simulink model "Nordic_2016a"  (R2016a)
settings: Solver=VariableStepAuto  StartTime=0.0  StopTime=600  RelTol=1e-3
values from neighbouring files (symbols this model uses):
  D = 10    [init_nordic.m]    (also in init_shj.m = 50)
  DC = [Y_11-Y_12*X*Y_21 Y_12*X]    [init_nordic.m]
  f0 = 50    [init_nordic.m]    (also in init_shj.m)
  H = [3.592 4.602 3.3 3.558 4.925 3.5 3.494 5.403 3.370 7]    [init_nordic.m]    (also in init_shj.m = 3)
  Kd1 = 0    [init_nordic.m]
  Kp = 2.5    [PID_parameters.m]    (also in init_nordic.m = 2)
  M1 = 5000    [init_nordic.m]    (also in init_shj.m = 300)
  M10 = 7800    [init_nordic.m]
  M2 = 6000    [init_nordic.m]    (also in init_shj.m = 30000)
  M3 = 8000    [init_nordic.m]
  M4 = 4400    [init_nordic.m]
  M5 = 14502    [init_nordic.m]
  M6 = 8000    [init_nordic.m]
  M7 = 2650    [init_nordic.m]
  M8 = 15300    [init_nordic.m]
  M9 = 11000    [init_nordic.m]
  Pl1 = 0    [init_nordic.m]
  Pl10 = 0    [init_nordic.m]
  Pl11 = 0    [init_nordic.m]
  Pl2 = 0    [init_nordic.m]
  Pl3 = 0    [init_nordic.m]
  Pl4 = 0    [init_nordic.m]
  Pl5 = 0    [init_nordic.m]
  Pl6 = 0    [init_nordic.m]
  Pl7 = 0.7    [init_nordic.m]
  Pl8 = 0    [init_nordic.m]
  Pl9 = 0    [init_nordic.m]
  R1 = 0.12    [init_nordic.m]
  R10 = 0.5    [init_nordic.m]
  R2 = R    (= 0.06)    [PID_parameters.m]    (also in init_nordic.m = 0.12)
  R3 = 0.12    [init_nordic.m]
  R4 = 0.12    [init_nordic.m]
  R5 = 0.25    [init_nordic.m]
  R6 = 0.12    [init_nordic.m]
  R7 = 0.12    [init_nordic.m]
  R8 = 0.5    [init_nordic.m]
  R9 = 0.12    [init_nordic.m]
  S_base = 1000    [init_nordic.m]    (also in init_shj.m = 30300)
  Td = 0.6    [PID_parameters.m]    (also in init_nordic.m = 0)
  Tf = 0.2    [PID_parameters.m]    (also in init_nordic.m = 0)
  Ti = 5    [PID_parameters.m]    (also in init_nordic.m)
  Tw = 1.5/2    (= 0.75)    [init_nordic.m]    (also in init_shj.m = 1.2)
  Ty = 0    [init_nordic.m]    (also in init_shj.m = 0.2)
  Ysp = 0    [init_nordic.m]    (also in init_shj.m)
settings Model: Creator=sigurd  LastModifiedBy=sigurdja

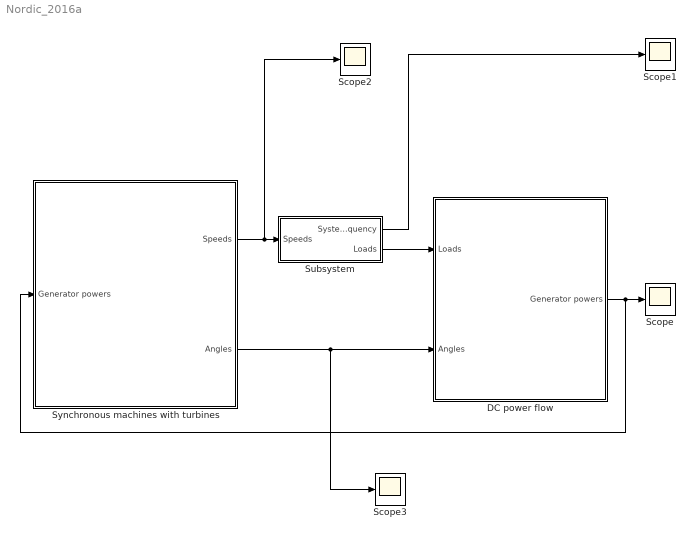
== system Nordic_2016a ==
  DC power flow : Subsystem
  Scope{,1..3} (4 alike) : Scope
  Subsystem : Subsystem
  Synchronous machines with turbines : Subsystem
  wires:
  DC power flow/1(Generator powers) -> Synchronous machines with turbines/1(Generator powers), Scope/1
  Synchronous machines with turbines/1(Speeds) -> Scope2/1, Subsystem/1(Speeds)
  Subsystem/2(Loads) -> DC power flow/1(Loads)
  Synchronous machines with turbines/2(Angles) -> Scope3/1, DC power flow/2(Angles)
  Subsystem/1(System frequency) -> Scope1/1

== system Nordic_2016a/DC power flow ==
  Loads : Inport
  Angles : Inport  Port=2
  Constant : Constant  Value=DC  VectorParams1D=off
  Demux : Demux  Outputs=10
  Demux1 : Demux  Outputs=11
  Gain : Gain  Gain=-1
  Mux : Mux  Inputs=21
  Product : Product  Multiplication=Matrix(*)
  Generator powers : Outport
  wires:
  Product/1 -> Generator powers/1
  Constant/1 -> Product/1
  Angles/1 -> Demux/1
  Loads/1 -> Gain/1
  Demux/1 -> Mux/1
  Demux/2 -> Mux/2
  Demux/3 -> Mux/3
  Demux/4 -> Mux/4
  Demux/5 -> Mux/5
  Demux/6 -> Mux/6
  Demux/7 -> Mux/7
  Demux/8 -> Mux/8
  Demux/9 -> Mux/9
  Demux/10 -> Mux/10
  Demux1/1 -> Mux/11
  Demux1/2 -> Mux/12
  Demux1/3 -> Mux/13
  Demux1/4 -> Mux/14
  Demux1/5 -> Mux/15
  Demux1/6 -> Mux/16
  Demux1/7 -> Mux/17
  Demux1/8 -> Mux/18
  Demux1/9 -> Mux/19
  Demux1/10 -> Mux/20
  Demux1/11 -> Mux/21
  Mux/1 -> Product/2
  Gain/1 -> Demux1/1

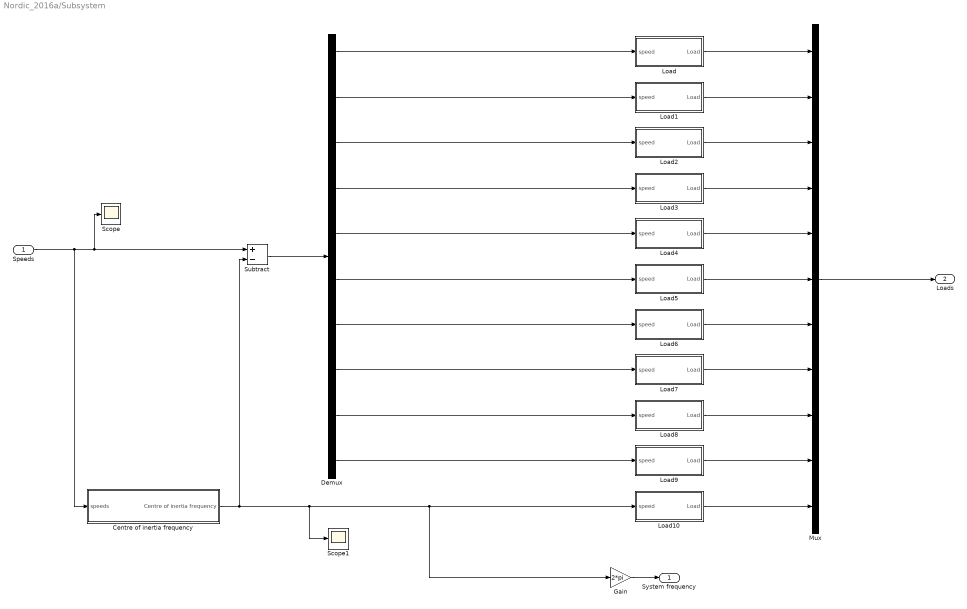
== system Nordic_2016a/Subsystem ==
  Speeds : Inport
  Centre of inertia frequency : Subsystem
  Demux : Demux  Outputs=10
  Gain : Gain  Gain=2*pi
  Load : Subsystem
  Load1 : Subsystem
  Load10 : Subsystem
  Load2 : Subsystem
  Load3 : Subsystem
  Load4 : Subsystem
  Load5 : Subsystem
  Load6 : Subsystem
  Load7 : Subsystem
  Load8 : Subsystem
  Load9 : Subsystem
  Mux : Mux  Inputs=11
  Scope : Scope
  Scope1 : Scope
  Subtract : Sum  Inputs=+-
  System frequency : Outport
  Loads : Outport  Port=2
  wires:
  Speeds/1 -> Centre of inertia frequency/1(speeds), Scope/1, Subtract/1
  Load/1(Load) -> Mux/1
  Load1/1(Load) -> Mux/2
  Load2/1(Load) -> Mux/3
  Load3/1(Load) -> Mux/4
  Load4/1(Load) -> Mux/5
  Load6/1(Load) -> Mux/7
  Load5/1(Load) -> Mux/6
  Load7/1(Load) -> Mux/8
  Load8/1(Load) -> Mux/9
  Mux/1 -> Loads/1
  Load9/1(Load) -> Mux/10
  Load10/1(Load) -> Mux/11
  Gain/1 -> System frequency/1
  Centre of inertia frequency/1(Centre of inertia frequency) -> Subtract/2, Scope1/1, Load10/1(speed), Gain/1
  Subtract/1 -> Demux/1
  Demux/1 -> Load/1(speed)
  Demux/2 -> Load1/1(speed)
  Demux/3 -> Load2/1(speed)
  Demux/4 -> Load3/1(speed)
  Demux/5 -> Load4/1(speed)
  Demux/6 -> Load5/1(speed)
  Demux/7 -> Load6/1(speed)
  Demux/8 -> Load7/1(speed)
  Demux/9 -> Load8/1(speed)
  Demux/10 -> Load9/1(speed)

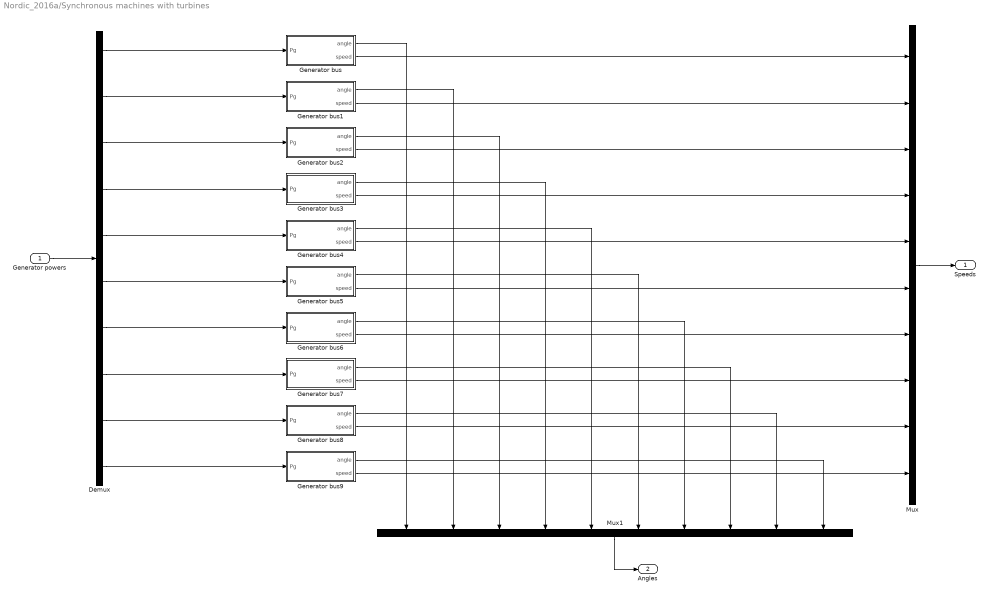
== system Nordic_2016a/Synchronous machines with turbines ==
  Generator powers : Inport  PortDimensions=10
  Demux : Demux  Outputs=10
  Generator bus : Subsystem
  Generator bus1 : Subsystem
  Generator bus2 : Subsystem
  Generator bus3 : Subsystem
  Generator bus4 : Subsystem
  Generator bus5 : Subsystem
  Generator bus6 : Subsystem
  Generator bus7 : Subsystem
  Generator bus8 : Subsystem
  Generator bus9 : Subsystem
  Mux : Mux  Inputs=10
  Mux1 : Mux  Inputs=10
  Speeds : Outport
  Angles : Outport  Port=2
  wires:
  Generator powers/1 -> Demux/1
  Demux/1 -> Generator bus/1(Pg)
  Demux/2 -> Generator bus1/1(Pg)
  Demux/3 -> Generator bus2/1(Pg)
  Demux/4 -> Generator bus3/1(Pg)
  Demux/5 -> Generator bus4/1(Pg)
  Demux/6 -> Generator bus5/1(Pg)
  Demux/7 -> Generator bus6/1(Pg)
  Demux/8 -> Generator bus7/1(Pg)
  Demux/9 -> Generator bus8/1(Pg)
  Demux/10 -> Generator bus9/1(Pg)
  Generator bus/1(angle) -> Mux1/1
  Generator bus1/1(angle) -> Mux1/2
  Generator bus2/1(angle) -> Mux1/3
  Generator bus3/1(angle) -> Mux1/4
  Generator bus4/1(angle) -> Mux1/5
  Generator bus5/1(angle) -> Mux1/6
  Generator bus6/1(angle) -> Mux1/7
  Generator bus7/1(angle) -> Mux1/8
  Generator bus8/1(angle) -> Mux1/9
  Generator bus9/1(angle) -> Mux1/10
  Mux1/1 -> Angles/1
  Generator bus/2(speed) -> Mux/1
  Generator bus1/2(speed) -> Mux/2
  Generator bus2/2(speed) -> Mux/3
  Generator bus3/2(speed) -> Mux/4
  Generator bus4/2(speed) -> Mux/5
  Generator bus5/2(speed) -> Mux/6
  Generator bus6/2(speed) -> Mux/7
  Generator bus7/2(speed) -> Mux/8
  Generator bus8/2(speed) -> Mux/9
  Generator bus9/2(speed) -> Mux/10
  Mux/1 -> Speeds/1

== system Nordic_2016a/Subsystem/Centre of inertia frequency ==
  speeds : Inport
  Add : Sum  Inputs=+
  Constant : Constant  Value=H  VectorParams1D=off
  Divide : Product  Inputs=/*
  Product : Product  Multiplication=Matrix(*)
  Centre of inertia frequency : Outport
  wires:
  Constant/1 -> Product/1, Add/1
  Product/1 -> Divide/2
  Add/1 -> Divide/1
  Divide/1 -> Centre of inertia frequency/1
  speeds/1 -> Product/2

== system Nordic_2016a/Subsystem/Load ==
  speed : Inport
  Gain : Gain  Gain=D
  Gain1 : Gain  Gain=M1/S_base
  Step : Step  After=Pl1  SampleTime=0
  Subtract : Sum  Inputs=-+
  Load : Outport
  wires:
  speed/1 -> Gain1/1
  Gain/1 -> Subtract/1
  Subtract/1 -> Load/1
  Step/1 -> Subtract/2
  Gain1/1 -> Gain/1

== system Nordic_2016a/Subsystem/Load1 ==
  speed : Inport
  Gain : Gain  Gain=D
  Gain1 : Gain  Gain=M2/S_base
  Step : Step  After=Pl2  SampleTime=0
  Subtract : Sum  Inputs=-+
  Load : Outport
  wires:
  speed/1 -> Gain1/1
  Gain/1 -> Subtract/1
  Subtract/1 -> Load/1
  Step/1 -> Subtract/2
  Gain1/1 -> Gain/1

== system Nordic_2016a/Subsystem/Load10 ==
  speed : Inport
  Step : Step  After=Pl11  SampleTime=0
  Subtract : Sum  Inputs=-+
  Load : Outport
  wires:
  Subtract/1 -> Load/1
  Step/1 -> Subtract/2

== system Nordic_2016a/Subsystem/Load2 ==
  speed : Inport
  Gain : Gain  Gain=D
  Gain1 : Gain  Gain=M3/S_base
  Step : Step  After=Pl3  SampleTime=0
  Subtract : Sum  Inputs=-+
  Load : Outport
  wires:
  speed/1 -> Gain1/1
  Gain/1 -> Subtract/1
  Subtract/1 -> Load/1
  Step/1 -> Subtract/2
  Gain1/1 -> Gain/1

== system Nordic_2016a/Subsystem/Load3 ==
  speed : Inport
  Gain : Gain  Gain=D
  Gain1 : Gain  Gain=M4/S_base
  Step : Step  After=Pl4  SampleTime=0
  Subtract : Sum  Inputs=-+
  Load : Outport
  wires:
  speed/1 -> Gain1/1
  Gain/1 -> Subtract/1
  Subtract/1 -> Load/1
  Step/1 -> Subtract/2
  Gain1/1 -> Gain/1

== system Nordic_2016a/Subsystem/Load4 ==
  speed : Inport
  Gain : Gain  Gain=D
  Gain1 : Gain  Gain=M5/S_base
  Step : Step  After=Pl5  SampleTime=0
  Subtract : Sum  Inputs=-+
  Load : Outport
  wires:
  speed/1 -> Gain1/1
  Gain/1 -> Subtract/1
  Subtract/1 -> Load/1
  Step/1 -> Subtract/2
  Gain1/1 -> Gain/1

== system Nordic_2016a/Subsystem/Load5 ==
  speed : Inport
  Gain : Gain  Gain=D
  Gain1 : Gain  Gain=M6/S_base
  Step : Step  After=Pl6  SampleTime=0
  Subtract : Sum  Inputs=-+
  Load : Outport
  wires:
  speed/1 -> Gain1/1
  Gain/1 -> Subtract/1
  Subtract/1 -> Load/1
  Step/1 -> Subtract/2
  Gain1/1 -> Gain/1

== system Nordic_2016a/Subsystem/Load6 ==
  speed : Inport
  Gain : Gain  Gain=D
  Gain1 : Gain  Gain=M7/S_base
  Step : Step  After=Pl7  SampleTime=0
  Subtract : Sum  Inputs=-+
  Load : Outport
  wires:
  speed/1 -> Gain1/1
  Gain/1 -> Subtract/1
  Subtract/1 -> Load/1
  Step/1 -> Subtract/2
  Gain1/1 -> Gain/1

== system Nordic_2016a/Subsystem/Load7 ==
  speed : Inport
  Gain : Gain  Gain=D
  Gain1 : Gain  Gain=M8/S_base
  Step : Step  After=Pl8  SampleTime=0
  Subtract : Sum  Inputs=-+
  Load : Outport
  wires:
  speed/1 -> Gain1/1
  Gain/1 -> Subtract/1
  Subtract/1 -> Load/1
  Step/1 -> Subtract/2
  Gain1/1 -> Gain/1

== system Nordic_2016a/Subsystem/Load8 ==
  speed : Inport
  Gain : Gain  Gain=D
  Gain1 : Gain  Gain=M9/S_base
  Step : Step  After=Pl9  SampleTime=0
  Subtract : Sum  Inputs=-+
  Load : Outport
  wires:
  speed/1 -> Gain1/1
  Gain/1 -> Subtract/1
  Subtract/1 -> Load/1
  Step/1 -> Subtract/2
  Gain1/1 -> Gain/1

== system Nordic_2016a/Subsystem/Load9 ==
  speed : Inport
  Gain : Gain  Gain=D
  Gain1 : Gain  Gain=M10/S_base
  Step : Step  After=Pl10  SampleTime=0
  Subtract : Sum  Inputs=-+
  Load : Outport
  wires:
  speed/1 -> Gain1/1
  Gain/1 -> Subtract/1
  Subtract/1 -> Load/1
  Step/1 -> Subtract/2
  Gain1/1 -> Gain/1

== system Nordic_2016a/Synchronous machines with turbines/Generator bus ==
  Pg : Inport
  Frequency dependent load5 : Gain  Gain=S_base/M1
  Frequency dependent load6 : Gain  Gain=2*pi*f0
  Governor1 : Subsystem
  Integrator1 : Integrator
  Sum3 : Sum  Inputs=|-+
  System inertia : TransferFcn  Denominator=[(2*H(1)) Kd1]
  angle : Outport
  speed : Outport  Port=2
  wires:
  Pg/1 -> Frequency dependent load5/1
  Governor1/1(u) -> Sum3/2
  Sum3/1 -> System inertia/1
  Frequency dependent load6/1 -> Integrator1/1
  System inertia/1 -> Governor1/1(Delta f), speed/1, Frequency dependent load6/1  "Change in frequency"
  Integrator1/1 -> angle/1
  Frequency dependent load5/1 -> Sum3/1

== system Nordic_2016a/Synchronous machines with turbines/Generator bus1 ==
  Pg : Inport
  Frequency dependent load5 : Gain  Gain=S_base/M2
  Frequency dependent load6 : Gain  Gain=2*pi*f0
  Governor1 : Subsystem
  Integrator1 : Integrator
  Sum3 : Sum  Inputs=|-+
  System inertia : TransferFcn  Denominator=[(2*H(2)) Kd1]
  angle : Outport
  speed : Outport  Port=2
  wires:
  Pg/1 -> Frequency dependent load5/1
  Governor1/1(u) -> Sum3/2
  Sum3/1 -> System inertia/1
  Frequency dependent load6/1 -> Integrator1/1
  System inertia/1 -> Governor1/1(Delta f), speed/1, Frequency dependent load6/1  "Change in frequency"
  Integrator1/1 -> angle/1
  Frequency dependent load5/1 -> Sum3/1

== system Nordic_2016a/Synchronous machines with turbines/Generator bus2 ==
  Pg : Inport
  Frequency dependent load5 : Gain  Gain=S_base/M3
  Frequency dependent load6 : Gain  Gain=2*pi*f0
  Governor1 : Subsystem
  Integrator1 : Integrator
  Sum3 : Sum  Inputs=|-+
  System inertia : TransferFcn  Denominator=[(2*H(3)) Kd1]
  angle : Outport
  speed : Outport  Port=2
  wires:
  Pg/1 -> Frequency dependent load5/1
  Governor1/1(u) -> Sum3/2
  Sum3/1 -> System inertia/1
  Frequency dependent load6/1 -> Integrator1/1
  System inertia/1 -> Governor1/1(Delta f), speed/1, Frequency dependent load6/1  "Change in frequency"
  Integrator1/1 -> angle/1
  Frequency dependent load5/1 -> Sum3/1

== system Nordic_2016a/Synchronous machines with turbines/Generator bus3 ==
  Pg : Inport
  Frequency dependent load5 : Gain  Gain=S_base/M4
  Frequency dependent load6 : Gain  Gain=2*pi*f0
  Governor1 : Subsystem
  Integrator1 : Integrator
  Sum3 : Sum  Inputs=|-+
  System inertia : TransferFcn  Denominator=[(2*H(4)) Kd1]
  angle : Outport
  speed : Outport  Port=2
  wires:
  Pg/1 -> Frequency dependent load5/1
  Governor1/1(u) -> Sum3/2
  Sum3/1 -> System inertia/1
  Frequency dependent load6/1 -> Integrator1/1
  System inertia/1 -> Governor1/1(Delta f), speed/1, Frequency dependent load6/1  "Change in frequency"
  Integrator1/1 -> angle/1
  Frequency dependent load5/1 -> Sum3/1

== system Nordic_2016a/Synchronous machines with turbines/Generator bus4 ==
  Pg : Inport
  Frequency dependent load5 : Gain  Gain=S_base/M5
  Frequency dependent load6 : Gain  Gain=2*pi*f0
  Governor1 : Subsystem
  Integrator1 : Integrator
  Sum3 : Sum  Inputs=|-+
  System inertia : TransferFcn  Denominator=[(2*H(5)) Kd1]
  angle : Outport
  speed : Outport  Port=2
  wires:
  Pg/1 -> Frequency dependent load5/1
  Governor1/1(u) -> Sum3/2
  Sum3/1 -> System inertia/1
  Frequency dependent load6/1 -> Integrator1/1
  System inertia/1 -> Governor1/1(Delta f), speed/1, Frequency dependent load6/1  "Change in frequency"
  Integrator1/1 -> angle/1
  Frequency dependent load5/1 -> Sum3/1

== system Nordic_2016a/Synchronous machines with turbines/Generator bus5 ==
  Pg : Inport
  Frequency dependent load5 : Gain  Gain=S_base/M6
  Frequency dependent load6 : Gain  Gain=2*pi*f0
  Governor1 : Subsystem
  Integrator1 : Integrator
  Sum3 : Sum  Inputs=|-+
  System inertia : TransferFcn  Denominator=[(2*H(6)) Kd1]
  angle : Outport
  speed : Outport  Port=2
  wires:
  Pg/1 -> Frequency dependent load5/1
  Governor1/1(u) -> Sum3/2
  Sum3/1 -> System inertia/1
  Frequency dependent load6/1 -> Integrator1/1
  System inertia/1 -> Governor1/1(Delta f), speed/1, Frequency dependent load6/1  "Change in frequency"
  Integrator1/1 -> angle/1
  Frequency dependent load5/1 -> Sum3/1

== system Nordic_2016a/Synchronous machines with turbines/Generator bus6 ==
  Pg : Inport
  Frequency dependent load5 : Gain  Gain=S_base/M7
  Frequency dependent load6 : Gain  Gain=2*pi*f0
  Governor1 : Subsystem
  Integrator1 : Integrator
  Sum3 : Sum  Inputs=|-+
  System inertia : TransferFcn  Denominator=[(2*H(7)) Kd1]
  angle : Outport
  speed : Outport  Port=2
  wires:
  Pg/1 -> Frequency dependent load5/1
  Governor1/1(u) -> Sum3/2
  Sum3/1 -> System inertia/1
  Frequency dependent load6/1 -> Integrator1/1
  System inertia/1 -> Governor1/1(Delta f), speed/1, Frequency dependent load6/1  "Change in frequency"
  Integrator1/1 -> angle/1
  Frequency dependent load5/1 -> Sum3/1

== system Nordic_2016a/Synchronous machines with turbines/Generator bus7 ==
  Pg : Inport
  Frequency dependent load5 : Gain  Gain=S_base/M8
  Frequency dependent load6 : Gain  Gain=2*pi*f0
  Governor1 : Subsystem
  Integrator1 : Integrator
  Sum3 : Sum  Inputs=|-+
  System inertia : TransferFcn  Denominator=[(2*H(8)) Kd1]
  angle : Outport
  speed : Outport  Port=2
  wires:
  Pg/1 -> Frequency dependent load5/1
  Governor1/1(u) -> Sum3/2
  Sum3/1 -> System inertia/1
  Frequency dependent load6/1 -> Integrator1/1
  System inertia/1 -> Governor1/1(Delta f), speed/1, Frequency dependent load6/1  "Change in frequency"
  Integrator1/1 -> angle/1
  Frequency dependent load5/1 -> Sum3/1

== system Nordic_2016a/Synchronous machines with turbines/Generator bus8 ==
  Pg : Inport
  Frequency dependent load5 : Gain  Gain=S_base/M9
  Frequency dependent load6 : Gain  Gain=2*pi*f0
  Governor1 : Subsystem
  Integrator1 : Integrator
  Sum3 : Sum  Inputs=|-+
  System inertia : TransferFcn  Denominator=[(2*H(9)) Kd1]
  angle : Outport
  speed : Outport  Port=2
  wires:
  Pg/1 -> Frequency dependent load5/1
  Governor1/1(u) -> Sum3/2
  Sum3/1 -> System inertia/1
  Frequency dependent load6/1 -> Integrator1/1
  System inertia/1 -> Governor1/1(Delta f), speed/1, Frequency dependent load6/1  "Change in frequency"
  Integrator1/1 -> angle/1
  Frequency dependent load5/1 -> Sum3/1

== system Nordic_2016a/Synchronous machines with turbines/Generator bus9 ==
  Pg : Inport
  Frequency dependent load5 : Gain  Gain=S_base/M10
  Frequency dependent load6 : Gain  Gain=2*pi*f0
  Governor1 : Subsystem
  Integrator1 : Integrator
  Sum3 : Sum  Inputs=|-+
  System inertia : TransferFcn  Denominator=[(2*H(10)) Kd1]
  angle : Outport
  speed : Outport  Port=2
  wires:
  Pg/1 -> Frequency dependent load5/1
  Governor1/1(u) -> Sum3/2
  Sum3/1 -> System inertia/1
  Frequency dependent load6/1 -> Integrator1/1
  System inertia/1 -> Governor1/1(Delta f), speed/1, Frequency dependent load6/1  "Change in frequency"
  Integrator1/1 -> angle/1
  Frequency dependent load5/1 -> Sum3/1

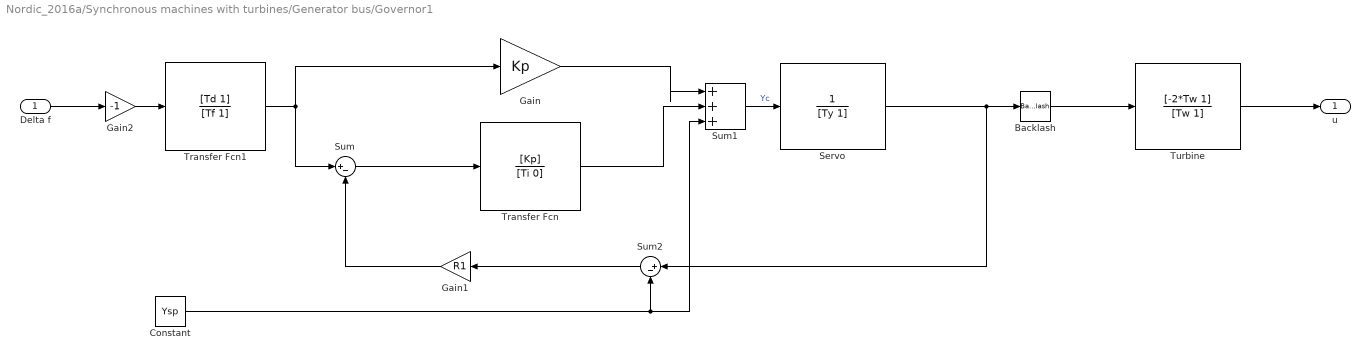
== system Nordic_2016a/Synchronous machines with turbines/Generator bus/Governor1 ==
  Delta f : Inport
  Backlash : Backlash  BacklashWidth=backlash
  Constant : Constant  Value=Ysp
  Gain : Gain  Gain=Kp
  Gain1 : Gain  Gain=R1
  Gain2 : Gain  Gain=-1
  Servo : TransferFcn  Denominator=[Ty 1]
  Sum : Sum  Inputs=|+-
  Sum1 : Sum  Inputs=|+++
  Sum2 : Sum  Inputs=|+-
  Transfer Fcn : TransferFcn  Numerator=[Kp]  Denominator=[Ti 0]
  Transfer Fcn1 : TransferFcn  Numerator=[Td 1]  Denominator=[Tf 1]
  Turbine : TransferFcn  Numerator=[-2*Tw 1]  Denominator=[Tw 1]
  u : Outport
  wires:
  Sum/1 -> Transfer Fcn/1
  Delta f/1 -> Gain2/1
  Gain/1 -> Sum1/1
  Transfer Fcn/1 -> Sum1/2
  Gain1/1 -> Sum/2
  Sum1/1 -> Servo/1  "Yc"
  Sum2/1 -> Gain1/1
  Constant/1 -> Sum1/3, Sum2/2
  Backlash/1 -> Turbine/1
  Turbine/1 -> u/1
  Gain2/1 -> Transfer Fcn1/1
  Transfer Fcn1/1 -> Gain/1, Sum/1
  Servo/1 -> Sum2/1, Backlash/1

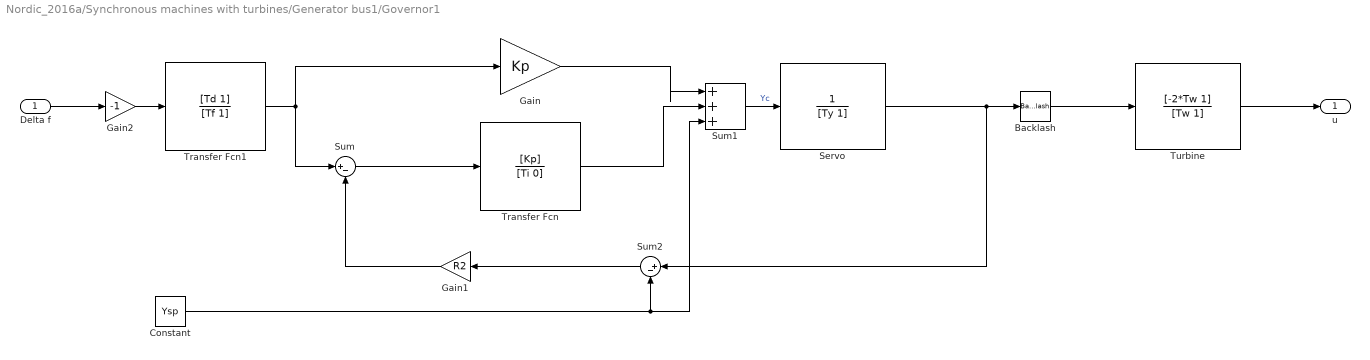
== system Nordic_2016a/Synchronous machines with turbines/Generator bus1/Governor1 ==
  Delta f : Inport
  Backlash : Backlash  BacklashWidth=backlash
  Constant : Constant  Value=Ysp
  Gain : Gain  Gain=Kp
  Gain1 : Gain  Gain=R2
  Gain2 : Gain  Gain=-1
  Servo : TransferFcn  Denominator=[Ty 1]
  Sum : Sum  Inputs=|+-
  Sum1 : Sum  Inputs=|+++
  Sum2 : Sum  Inputs=|+-
  Transfer Fcn : TransferFcn  Numerator=[Kp]  Denominator=[Ti 0]
  Transfer Fcn1 : TransferFcn  Numerator=[Td 1]  Denominator=[Tf 1]
  Turbine : TransferFcn  Numerator=[-2*Tw 1]  Denominator=[Tw 1]
  u : Outport
  wires:
  Sum/1 -> Transfer Fcn/1
  Delta f/1 -> Gain2/1
  Gain/1 -> Sum1/1
  Transfer Fcn/1 -> Sum1/2
  Gain1/1 -> Sum/2
  Sum1/1 -> Servo/1  "Yc"
  Sum2/1 -> Gain1/1
  Constant/1 -> Sum1/3, Sum2/2
  Backlash/1 -> Turbine/1
  Turbine/1 -> u/1
  Gain2/1 -> Transfer Fcn1/1
  Transfer Fcn1/1 -> Gain/1, Sum/1
  Servo/1 -> Sum2/1, Backlash/1

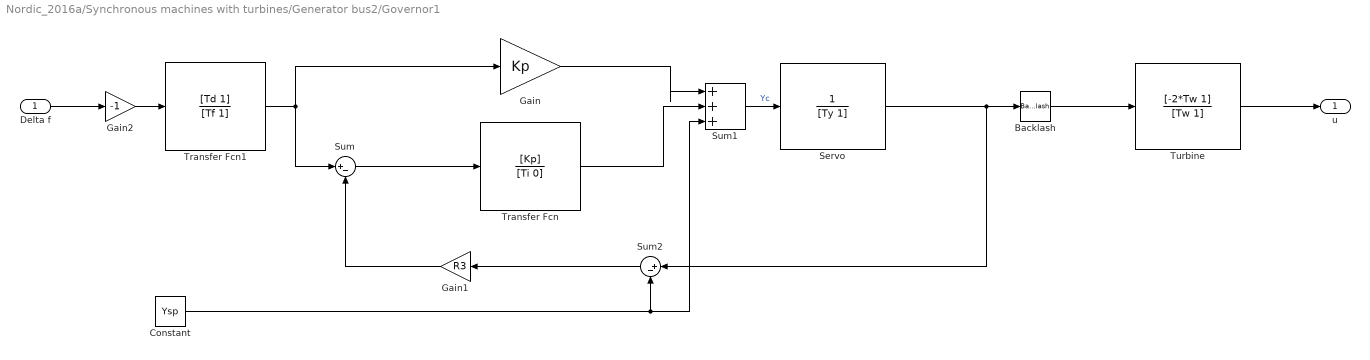
== system Nordic_2016a/Synchronous machines with turbines/Generator bus2/Governor1 ==
  Delta f : Inport
  Backlash : Backlash  BacklashWidth=backlash
  Constant : Constant  Value=Ysp
  Gain : Gain  Gain=Kp
  Gain1 : Gain  Gain=R3
  Gain2 : Gain  Gain=-1
  Servo : TransferFcn  Denominator=[Ty 1]
  Sum : Sum  Inputs=|+-
  Sum1 : Sum  Inputs=|+++
  Sum2 : Sum  Inputs=|+-
  Transfer Fcn : TransferFcn  Numerator=[Kp]  Denominator=[Ti 0]
  Transfer Fcn1 : TransferFcn  Numerator=[Td 1]  Denominator=[Tf 1]
  Turbine : TransferFcn  Numerator=[-2*Tw 1]  Denominator=[Tw 1]
  u : Outport
  wires:
  Sum/1 -> Transfer Fcn/1
  Delta f/1 -> Gain2/1
  Gain/1 -> Sum1/1
  Transfer Fcn/1 -> Sum1/2
  Gain1/1 -> Sum/2
  Sum1/1 -> Servo/1  "Yc"
  Sum2/1 -> Gain1/1
  Constant/1 -> Sum1/3, Sum2/2
  Backlash/1 -> Turbine/1
  Turbine/1 -> u/1
  Gain2/1 -> Transfer Fcn1/1
  Transfer Fcn1/1 -> Gain/1, Sum/1
  Servo/1 -> Sum2/1, Backlash/1

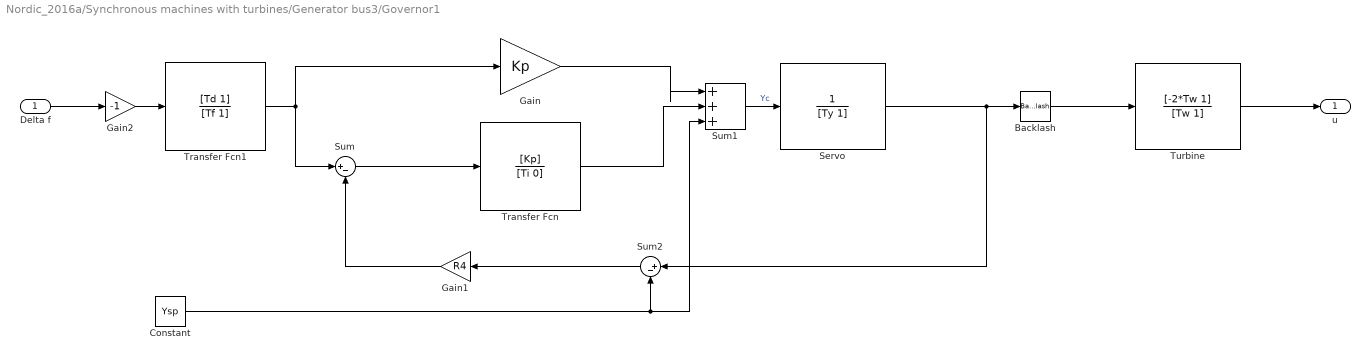
== system Nordic_2016a/Synchronous machines with turbines/Generator bus3/Governor1 ==
  Delta f : Inport
  Backlash : Backlash  BacklashWidth=backlash
  Constant : Constant  Value=Ysp
  Gain : Gain  Gain=Kp
  Gain1 : Gain  Gain=R4
  Gain2 : Gain  Gain=-1
  Servo : TransferFcn  Denominator=[Ty 1]
  Sum : Sum  Inputs=|+-
  Sum1 : Sum  Inputs=|+++
  Sum2 : Sum  Inputs=|+-
  Transfer Fcn : TransferFcn  Numerator=[Kp]  Denominator=[Ti 0]
  Transfer Fcn1 : TransferFcn  Numerator=[Td 1]  Denominator=[Tf 1]
  Turbine : TransferFcn  Numerator=[-2*Tw 1]  Denominator=[Tw 1]
  u : Outport
  wires:
  Sum/1 -> Transfer Fcn/1
  Delta f/1 -> Gain2/1
  Gain/1 -> Sum1/1
  Transfer Fcn/1 -> Sum1/2
  Gain1/1 -> Sum/2
  Sum1/1 -> Servo/1  "Yc"
  Sum2/1 -> Gain1/1
  Constant/1 -> Sum1/3, Sum2/2
  Backlash/1 -> Turbine/1
  Turbine/1 -> u/1
  Gain2/1 -> Transfer Fcn1/1
  Transfer Fcn1/1 -> Gain/1, Sum/1
  Servo/1 -> Sum2/1, Backlash/1

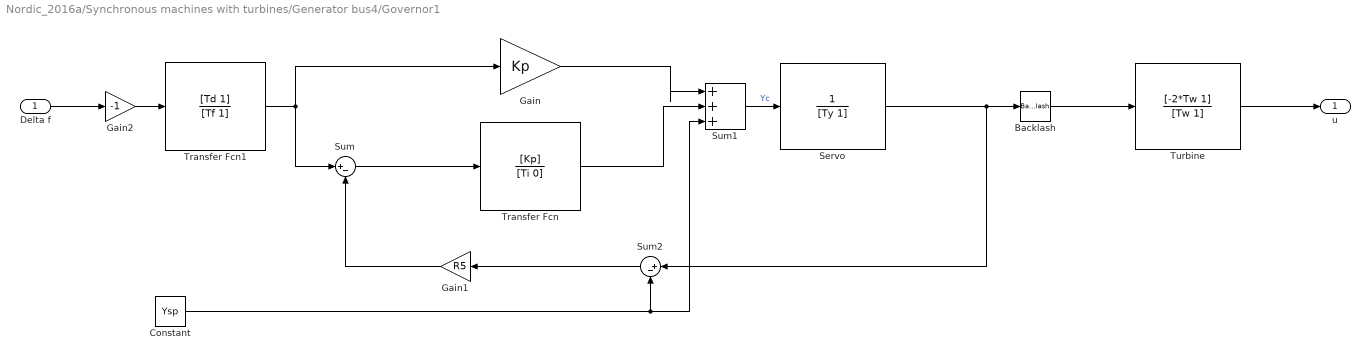
== system Nordic_2016a/Synchronous machines with turbines/Generator bus4/Governor1 ==
  Delta f : Inport
  Backlash : Backlash  BacklashWidth=backlash
  Constant : Constant  Value=Ysp
  Gain : Gain  Gain=Kp
  Gain1 : Gain  Gain=R5
  Gain2 : Gain  Gain=-1
  Servo : TransferFcn  Denominator=[Ty 1]
  Sum : Sum  Inputs=|+-
  Sum1 : Sum  Inputs=|+++
  Sum2 : Sum  Inputs=|+-
  Transfer Fcn : TransferFcn  Numerator=[Kp]  Denominator=[Ti 0]
  Transfer Fcn1 : TransferFcn  Numerator=[Td 1]  Denominator=[Tf 1]
  Turbine : TransferFcn  Numerator=[-2*Tw 1]  Denominator=[Tw 1]
  u : Outport
  wires:
  Sum/1 -> Transfer Fcn/1
  Delta f/1 -> Gain2/1
  Gain/1 -> Sum1/1
  Transfer Fcn/1 -> Sum1/2
  Gain1/1 -> Sum/2
  Sum1/1 -> Servo/1  "Yc"
  Sum2/1 -> Gain1/1
  Constant/1 -> Sum1/3, Sum2/2
  Backlash/1 -> Turbine/1
  Turbine/1 -> u/1
  Gain2/1 -> Transfer Fcn1/1
  Transfer Fcn1/1 -> Gain/1, Sum/1
  Servo/1 -> Sum2/1, Backlash/1

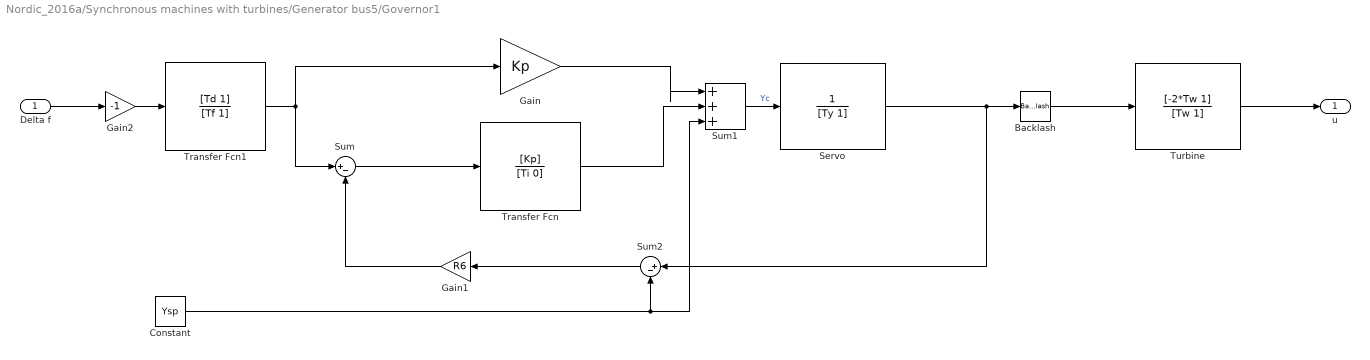
== system Nordic_2016a/Synchronous machines with turbines/Generator bus5/Governor1 ==
  Delta f : Inport
  Backlash : Backlash  BacklashWidth=backlash
  Constant : Constant  Value=Ysp
  Gain : Gain  Gain=Kp
  Gain1 : Gain  Gain=R6
  Gain2 : Gain  Gain=-1
  Servo : TransferFcn  Denominator=[Ty 1]
  Sum : Sum  Inputs=|+-
  Sum1 : Sum  Inputs=|+++
  Sum2 : Sum  Inputs=|+-
  Transfer Fcn : TransferFcn  Numerator=[Kp]  Denominator=[Ti 0]
  Transfer Fcn1 : TransferFcn  Numerator=[Td 1]  Denominator=[Tf 1]
  Turbine : TransferFcn  Numerator=[-2*Tw 1]  Denominator=[Tw 1]
  u : Outport
  wires:
  Sum/1 -> Transfer Fcn/1
  Delta f/1 -> Gain2/1
  Gain/1 -> Sum1/1
  Transfer Fcn/1 -> Sum1/2
  Gain1/1 -> Sum/2
  Sum1/1 -> Servo/1  "Yc"
  Sum2/1 -> Gain1/1
  Constant/1 -> Sum1/3, Sum2/2
  Backlash/1 -> Turbine/1
  Turbine/1 -> u/1
  Gain2/1 -> Transfer Fcn1/1
  Transfer Fcn1/1 -> Gain/1, Sum/1
  Servo/1 -> Sum2/1, Backlash/1

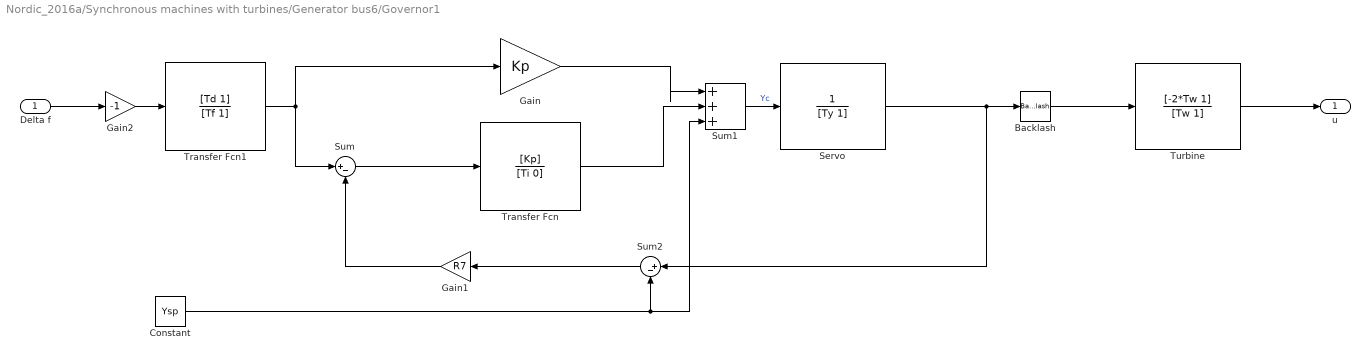
== system Nordic_2016a/Synchronous machines with turbines/Generator bus6/Governor1 ==
  Delta f : Inport
  Backlash : Backlash  BacklashWidth=backlash
  Constant : Constant  Value=Ysp
  Gain : Gain  Gain=Kp
  Gain1 : Gain  Gain=R7
  Gain2 : Gain  Gain=-1
  Servo : TransferFcn  Denominator=[Ty 1]
  Sum : Sum  Inputs=|+-
  Sum1 : Sum  Inputs=|+++
  Sum2 : Sum  Inputs=|+-
  Transfer Fcn : TransferFcn  Numerator=[Kp]  Denominator=[Ti 0]
  Transfer Fcn1 : TransferFcn  Numerator=[Td 1]  Denominator=[Tf 1]
  Turbine : TransferFcn  Numerator=[-2*Tw 1]  Denominator=[Tw 1]
  u : Outport
  wires:
  Sum/1 -> Transfer Fcn/1
  Delta f/1 -> Gain2/1
  Gain/1 -> Sum1/1
  Transfer Fcn/1 -> Sum1/2
  Gain1/1 -> Sum/2
  Sum1/1 -> Servo/1  "Yc"
  Sum2/1 -> Gain1/1
  Constant/1 -> Sum1/3, Sum2/2
  Backlash/1 -> Turbine/1
  Turbine/1 -> u/1
  Gain2/1 -> Transfer Fcn1/1
  Transfer Fcn1/1 -> Gain/1, Sum/1
  Servo/1 -> Sum2/1, Backlash/1

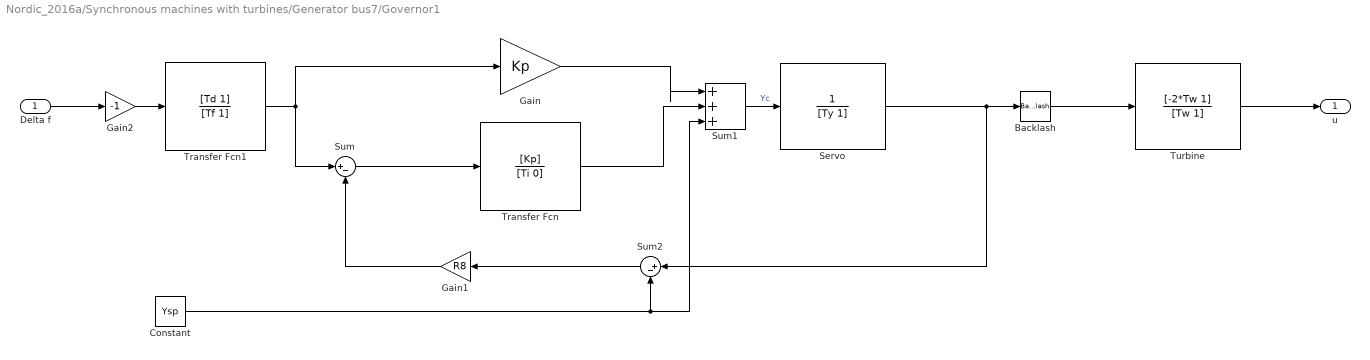
== system Nordic_2016a/Synchronous machines with turbines/Generator bus7/Governor1 ==
  Delta f : Inport
  Backlash : Backlash  BacklashWidth=backlash
  Constant : Constant  Value=Ysp
  Gain : Gain  Gain=Kp
  Gain1 : Gain  Gain=R8
  Gain2 : Gain  Gain=-1
  Servo : TransferFcn  Denominator=[Ty 1]
  Sum : Sum  Inputs=|+-
  Sum1 : Sum  Inputs=|+++
  Sum2 : Sum  Inputs=|+-
  Transfer Fcn : TransferFcn  Numerator=[Kp]  Denominator=[Ti 0]
  Transfer Fcn1 : TransferFcn  Numerator=[Td 1]  Denominator=[Tf 1]
  Turbine : TransferFcn  Numerator=[-2*Tw 1]  Denominator=[Tw 1]
  u : Outport
  wires:
  Sum/1 -> Transfer Fcn/1
  Delta f/1 -> Gain2/1
  Gain/1 -> Sum1/1
  Transfer Fcn/1 -> Sum1/2
  Gain1/1 -> Sum/2
  Sum1/1 -> Servo/1  "Yc"
  Sum2/1 -> Gain1/1
  Constant/1 -> Sum1/3, Sum2/2
  Backlash/1 -> Turbine/1
  Turbine/1 -> u/1
  Gain2/1 -> Transfer Fcn1/1
  Transfer Fcn1/1 -> Gain/1, Sum/1
  Servo/1 -> Sum2/1, Backlash/1

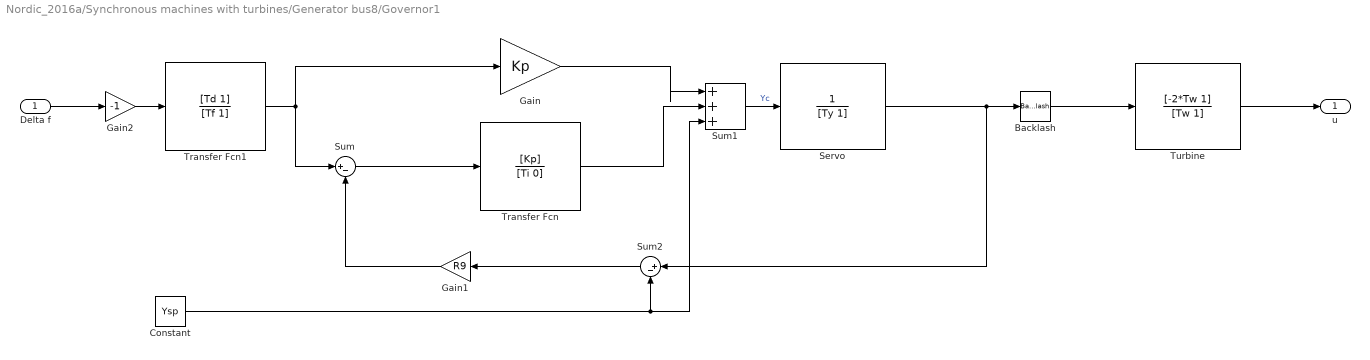
== system Nordic_2016a/Synchronous machines with turbines/Generator bus8/Governor1 ==
  Delta f : Inport
  Backlash : Backlash  BacklashWidth=backlash
  Constant : Constant  Value=Ysp
  Gain : Gain  Gain=Kp
  Gain1 : Gain  Gain=R9
  Gain2 : Gain  Gain=-1
  Servo : TransferFcn  Denominator=[Ty 1]
  Sum : Sum  Inputs=|+-
  Sum1 : Sum  Inputs=|+++
  Sum2 : Sum  Inputs=|+-
  Transfer Fcn : TransferFcn  Numerator=[Kp]  Denominator=[Ti 0]
  Transfer Fcn1 : TransferFcn  Numerator=[Td 1]  Denominator=[Tf 1]
  Turbine : TransferFcn  Numerator=[-2*Tw 1]  Denominator=[Tw 1]
  u : Outport
  wires:
  Sum/1 -> Transfer Fcn/1
  Delta f/1 -> Gain2/1
  Gain/1 -> Sum1/1
  Transfer Fcn/1 -> Sum1/2
  Gain1/1 -> Sum/2
  Sum1/1 -> Servo/1  "Yc"
  Sum2/1 -> Gain1/1
  Constant/1 -> Sum1/3, Sum2/2
  Backlash/1 -> Turbine/1
  Turbine/1 -> u/1
  Gain2/1 -> Transfer Fcn1/1
  Transfer Fcn1/1 -> Gain/1, Sum/1
  Servo/1 -> Sum2/1, Backlash/1

== system Nordic_2016a/Synchronous machines with turbines/Generator bus9/Governor1 ==
  Delta f : Inport
  Backlash : Backlash  BacklashWidth=backlash
  Constant : Constant  Value=Ysp
  Gain : Gain  Gain=Kp
  Gain1 : Gain  Gain=R10
  Gain2 : Gain  Gain=-1
  Servo : TransferFcn  Denominator=[Ty 1]
  Sum : Sum  Inputs=|+-
  Sum1 : Sum  Inputs=|+++
  Sum2 : Sum  Inputs=|+-
  Transfer Fcn : TransferFcn  Numerator=[Kp]  Denominator=[Ti 0]
  Transfer Fcn1 : TransferFcn  Numerator=[Td 1]  Denominator=[Tf 1]
  Turbine : TransferFcn  Numerator=[-2*Tw 1]  Denominator=[Tw 1]
  u : Outport
  wires:
  Sum/1 -> Transfer Fcn/1
  Delta f/1 -> Gain2/1
  Gain/1 -> Sum1/1
  Transfer Fcn/1 -> Sum1/2
  Gain1/1 -> Sum/2
  Sum1/1 -> Servo/1  "Yc"
  Sum2/1 -> Gain1/1
  Constant/1 -> Sum1/3, Sum2/2
  Backlash/1 -> Turbine/1
  Turbine/1 -> u/1
  Gain2/1 -> Transfer Fcn1/1
  Transfer Fcn1/1 -> Gain/1, Sum/1
  Servo/1 -> Sum2/1, Backlash/1
